simulink model "euler_angles_to_quaternions"  (R2023a)
settings: Solver=VariableStepAuto  StartTime=0.0  StopTime=50  RelTol=1e-3
settings Model: Creator=ganes  LastModifiedBy=ganes

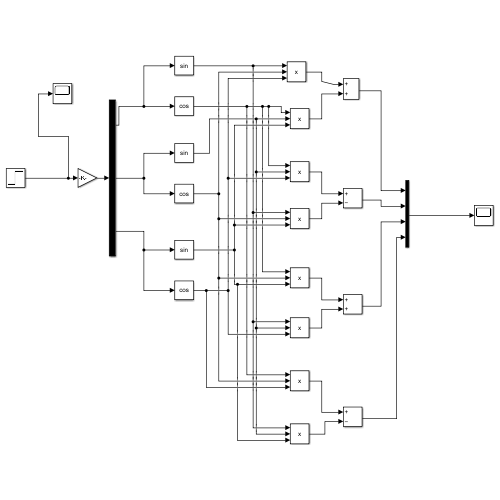
[thumbnail: Simulink's stored preview of the top-level diagram]
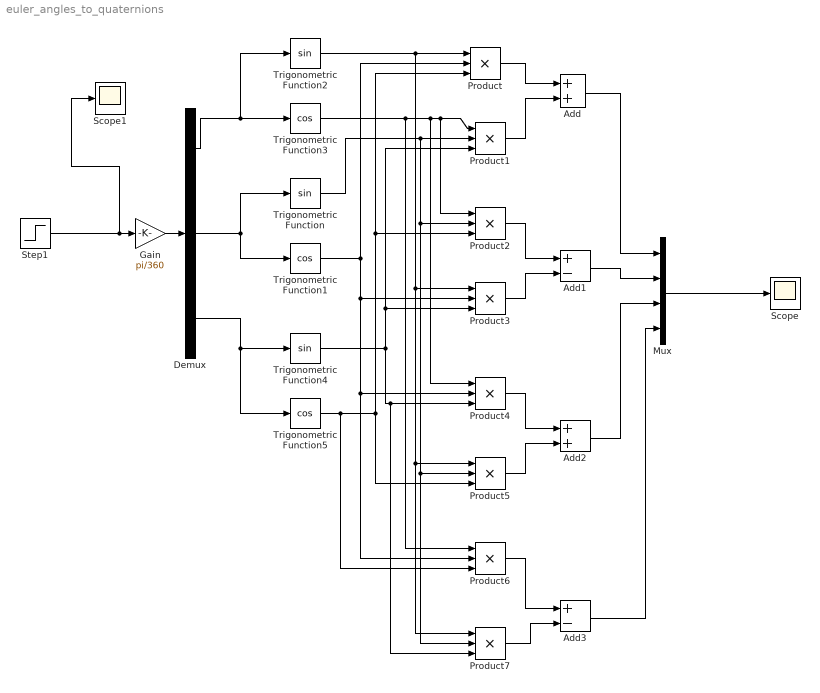
== system euler_angles_to_quaternions ==
  Add : Sum
  Add1 : Sum  Inputs=+-
  Add2 : Sum
  Add3 : Sum  Inputs=+-
  Demux : Demux  Outputs=3
  Gain : Gain  Gain=pi/360
  Mux : Mux
  Product{,1..7} (8 alike) : Product  Inputs=3  RndMeth=Zero
  Scope : Scope
  Scope1 : Scope
  Step1 : Step  Time=40  Before=[20 -10 30]  After="[45 -25  15]"  SampleTime=0
  Trigonometric Function : Trigonometry
  Trigonometric Function1 : Trigonometry  Operator=cos
  Trigonometric Function2 : Trigonometry
  Trigonometric Function3 : Trigonometry  Operator=cos
  Trigonometric Function4 : Trigonometry
  Trigonometric Function5 : Trigonometry  Operator=cos
  wires:
  Gain/1 -> Demux/1
  Add3/1 -> Mux/4
  Add2/1 -> Mux/3
  Product6/1 -> Add3/1
  Add1/1 -> Mux/2
  Product/1 -> Add/1
  Product4/1 -> Add2/1
  Trigonometric Function5/1 -> Product/3, Product2/3, Product5/3, Product6/3
  Demux/1 -> Trigonometric Function2/1, Trigonometric Function3/1
  Product1/1 -> Add/2
  Step1/1 -> Scope1/1, Gain/1
  Trigonometric Function1/1 -> Product/2, Product3/2, Product4/2, Product6/2
  Product7/1 -> Add3/2
  Trigonometric Function/1 -> Product1/2, Product2/2, Product5/2, Product7/2
  Demux/3 -> Trigonometric Function4/1, Trigonometric Function5/1
  Mux/1 -> Scope/1
  Trigonometric Function2/1 -> Product/1, Product3/1, Product5/1, Product7/1
  Trigonometric Function4/1 -> Product1/3, Product3/3, Product4/3, Product7/3
  Trigonometric Function3/1 -> Product1/1, Product2/1, Product4/1, Product6/1
  Add/1 -> Mux/1
  Product5/1 -> Add2/2
  Demux/2 -> Trigonometric Function/1, Trigonometric Function1/1
  Product3/1 -> Add1/2
  Product2/1 -> Add1/1
